simulink model "levitacao2"  (R2013a)
settings: Solver=FixedStepDiscrete  StartTime=0.0  StopTime=inf  RelTol=1e-3
undefined symbols (not defined in the file): DiscIntNeverNeededParam
libraries: arduino_io_lib x10, simulink x10
settings Model: Creator=gcampa  LastModifiedBy=Felipe
settings DataIOCC: SignalLoggingSaveFormat=ModelDataLogs
settings OptimizationCC: ExpressionDepthLimit=2147483647
settings DebuggingCC: FcnCallInpInsideContextMsg=UseLocalSettings
settings GRTTargetCC: CombineOutputUpdateFcns=off  GRTInterface=on

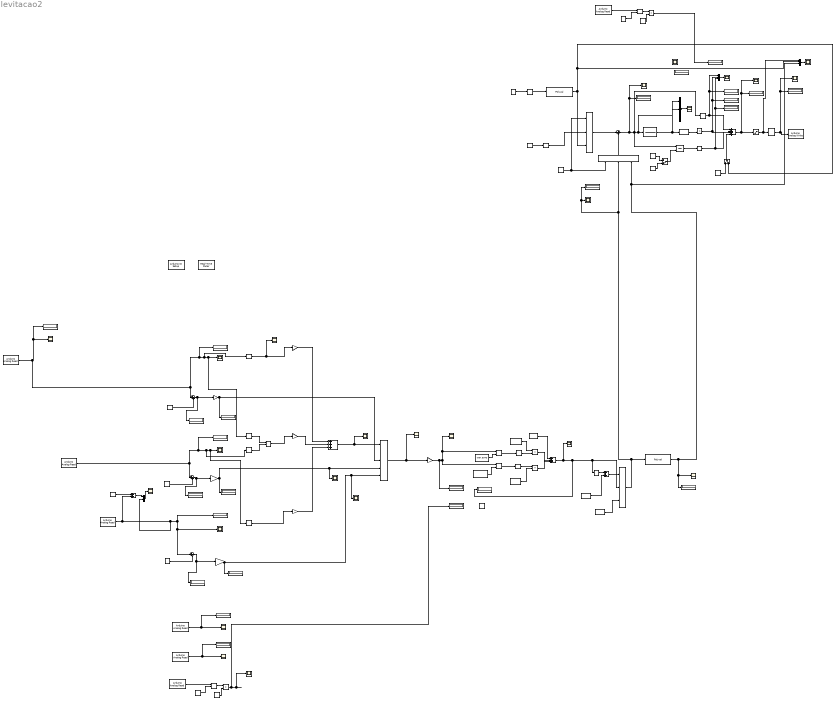
== system levitacao2 ==
  note: tem relacao com a distancia
  note: 0 para escolher realimentação do sinal de distancia cm
      | 1 para escolher sinal de realimentacao do sinal pwm0
  note: pwm0 ref
  note: funçao pwm0 X posicao(cm)
  note: bias - pwm0
  note: Funcao PWM0 X posicao0(cm)
  note: posicao em cm
  note: erro
  note: Set point ou distancia desejada em cm
  note: Distancia em cm
  note: Lê o potenciometro e envia para a saida pwm
  note: Sinal dos 3 sensores em 1 - sinal processado
  note: Converte sinal do sensor para distancia em cm - equação de decaimento exponencial de ordem 2
  note: se 1 - escolhe sensor 1
      | se 2 - escolhe sensor 2
      | se 3 - escolhe sensor 3
  note: Selecionando o sensor de acordo com sua sensibilidade para uma determinada faixa
  note: Tirando o ganho do amplificador
  note: Tirando o offset do circuito amplificador
  note: Tirando o offset do circuito amplificador
  note: Tirando o offset do circuito amplificador
  note: Tirando o ganho do amplificador
  note: Tirando o ganho do amplificador
  note: Selecionando o sensor de acordo com sua sensibilidade para uma determinada faixa
  note: Selecionando o sensor de acordo com sua sensibilidade para uma determinada faixa
  note: Set point ou distancia desejada em cm
  Add : Sum  Inputs=+++
  Add1 : Sum  Inputs=++++
  Add2 : Sum
  Arduino Analog Read16 : arduino_io_lib/Arduino Analog Read  arduinoVar=Temporary arduino variable: Arduino1  arduinoPin=1  T=0.00002
  Arduino Analog Read2 : arduino_io_lib/Arduino Analog Read  arduinoVar=Temporary arduino variable: Arduino1  arduinoPin=0  T=0.00002
  Arduino Analog Read3 : arduino_io_lib/Arduino Analog Read  arduinoVar=Temporary arduino variable: Arduino1  arduinoPin=3  T=0.00002
  Arduino Analog Read4 : arduino_io_lib/Arduino Analog Read  arduinoVar=Temporary arduino variable: Arduino1  arduinoPin=2  T=0.00002
  Arduino Analog Read5 : arduino_io_lib/Arduino Analog Read  arduinoVar=Temporary arduino variable: Arduino1  arduinoPin=2  T=0.001
  Arduino Analog Read6 : arduino_io_lib/Arduino Analog Read  arduinoVar=Temporary arduino variable: Arduino1  arduinoPin=4  T=0.01
  Arduino Analog Read7 : arduino_io_lib/Arduino Analog Read  arduinoVar=Temporary arduino variable: Arduino1  arduinoPin=3  T=0.001
  Arduino Analog Write3 : arduino_io_lib/Arduino Analog Write  arduinoVar=Temporary arduino variable: Arduino1  arduinoPin=5  T=0.00001
  Arduino IO Setup : arduino_io_lib/Arduino IO Setup  Priority=3  arduinoVar=Temporary arduino variable: Arduino1  workspaceVarName=a  comPort=COM3
  Compare To Constant : simulink/Logic and Bit Operations/Compare To Constant  relop=>=  const=56  OutDataTypeStr=boolean
  Compare To Constant1 : simulink/Logic and Bit Operations/Compare To Constant  relop=<  const=56  OutDataTypeStr=boolean
  Compare To Constant2 : simulink/Logic and Bit Operations/Compare To Constant  relop=>=  const=165  OutDataTypeStr=boolean
  Compare To Constant3 : simulink/Logic and Bit Operations/Compare To Constant  relop=<  const=160  OutDataTypeStr=boolean
  Compare To Constant4 : simulink/Logic and Bit Operations/Compare To Constant  relop=>  const=4  OutDataTypeStr=boolean
  Constant10 : Constant  Value=3.96648
  Constant11 : Constant  Value=0.01226
  Constant12 : Constant  Value=-56.90857
  Constant{9,13..16} (5 alike) : Constant
  Constant17 : Constant  Value=0
  Constant18 : Constant  Value=10
  Constant19 : Constant  Value=0
  Constant2 : Constant  Value=100
  Constant20 : Constant  Value=4
  Constant21 : Constant  Value=1023
  Constant22 : Constant  Value=0
  Constant23 : Constant  Value=0.00001
  Constant3 : Constant  Value=5
  Constant4 : Constant  Value=400
  Constant5 : Constant  Value=1023
  Constant6 : Constant  Value=256
  Constant7 : Constant  Value=2.24554
  Constant8 : Constant  Value=-587.5943
  Discrete Derivative : simulink/Discrete/Discrete Derivative  gainval=1.0  ICPrevScaledInput=0.0  InputProcessing=Inherited  OutMin=[]  OutMax=[]  OutDataType=fixdt(1, 16)  OutScaling=2^-10  DoSatur=off
  Discrete Filter1 : DiscreteFilter  Numerator=[0.5 0.5]  Denominator=[1 0.00001]  InputProcessing=Columns as channels (frame based)  FilterStructure=Direct form II transposed  a0EqualsOne=on
  Discrete-Time Integrator : DiscreteIntegrator  ExternalReset=either  SampleTime=0.00002  ICPrevOutput=DiscIntNeverNeededParam  ICPrevScaledInput=DiscIntNeverNeededParam
  Display{,1..24} (25 alike) : Display
  Divide{,1..3} (4 alike) : Product  Inputs=*/
  Gain : Gain
  Gain1 : Gain  Gain=2
  Gain2 : Gain  Gain=3
  Gain3 : Gain
  Gain4 : Gain  Gain=0.094
  Gain5 : Gain  Gain=0.024
  Gain6 : Gain  Gain=10
  Logical Operator : Logic  AllPortsSameDT=off  OutDataTypeStr=boolean
  Manual Switch : ManualSwitch  CurrentSetting=0
  Manual Switch1 : ManualSwitch  CurrentSetting=0
  Math Function : Math  SaturateOnIntegerOverflow=on
  Math Function1 : Math  SaturateOnIntegerOverflow=on
  Mode Multiport Switch : MultiPortSwitch  DataPortOrder=Zero-based contiguous  Inputs=4  zeroidx=on
  Mode Multiport Switch1 : MultiPortSwitch  DataPortOrder=Zero-based contiguous  Inputs=2  zeroidx=on
  Mode Multiport Switch2 : MultiPortSwitch  DataPortOrder=Zero-based contiguous  Inputs=2  zeroidx=on
  Mode Multiport Switch3 : MultiPortSwitch  DataPortOrder=Zero-based contiguous  Inputs=2  zeroidx=on
  Mux1 : Mux
      settings: DisplayOption=signals
  Mux2 : Mux  Inputs=2
      settings: DisplayOption=signals
  Mux3 : Mux
      settings: DisplayOption=signals
  Mux4 : Mux  Inputs=3
      settings: DisplayOption=signals
  Polynomial : Polyval  Coefs=[11.55, 16.03, 27.7 ]
  Polynomial1 : Polyval  Coefs=[11.55, 16.03, 27.7 ]
  Product{,1,3..5} (5 alike) : Product
  Rate Transition : RateTransition
  Real-Time Pacer : arduino_io_lib/Real-Time Pacer  simTimePerRealTime=1
  Saturation : Saturate  UpperLimit=255  LowerLimit=0
      settings: AttributesFormatString=max = %<UpperLimit>\nmin = %<LowerLimit>
  Scope{1..24} (24 alike) : Scope
      Scope1 settings: YMin=41  YMax=43.2
      Scope10 settings: YMin=0  YMax=1023  SaveName=ScopeData10
      Scope11 settings: YMin=4.25  YMax=8  SaveName=ScopeData11
      Scope12 settings: YMin=0  YMax=1023  SaveName=ScopeData12
      Scope13 settings: YMin=0  YMax=1023  SaveName=ScopeData13
      Scope14 settings: TimeRange=1  YMin=1  YMax=6.25  SaveName=ScopeData14
      Scope15 settings: YMin=-6  YMax=2  SaveName=ScopeData15
      Scope16 settings: TimeRange=0.1  YMin=80  YMax=155  SaveName=ScopeData16
      Scope17 settings: YMin=170.66  YMax=170.66  SaveName=ScopeData17
      Scope18 settings: TimeRange=1e-05  YMin=-75  YMax=250  SaveName=ScopeData18
      Scope19 settings: YMin=50  YMax=1100  SaveName=ScopeData19
      Scope2 settings: YMin=0  YMax=1023  SaveName=ScopeData2
      Scope20 settings: TimeRange=0.3  YMin=0  YMax=275  SaveName=ScopeData20
      Scope21 settings: TimeRange=1e-05  YMin=320  YMax=550  SaveName=ScopeData21
      Scope22 settings: YMin=2.5  YMax=50  SaveName=ScopeData22
      Scope23 settings: TimeRange=0.05  YMin=0  YMax=300  SaveName=ScopeData23
      Scope24 settings: TimeRange=0.01  YMin=0  YMax=180  SaveName=ScopeData24
      Scope3 settings: YMin=0  YMax=1023  SaveName=ScopeData3
      Scope4 settings: YMin=0  YMax=1023  SaveName=ScopeData4
      Scope5 settings: YMin=0  YMax=1023  SaveName=ScopeData5
      Scope6 settings: YMin=0  YMax=1023  SaveName=ScopeData6
      Scope7 settings: YMin=0  YMax=1023  SaveName=ScopeData7
      Scope8 settings: YMin=0  YMax=1023  SaveName=ScopeData8
      Scope9 settings: TimeRange=1  YMin=-2.5  YMax=27.5  SaveName=ScopeData9
  Slider Gain2 : simulink/Math Operations/Slider Gain  low=0  gain=2.5  high=3.6
  Slider Gain3 : simulink/Math Operations/Slider Gain  low=0  gain=1.24  high=2
  Slider Gain5 : simulink/Math Operations/Slider Gain  low=0  gain=0  high=100
  Slider Gain6 : simulink/Math Operations/Slider Gain  low=0  gain=2  high=3.6
  Subtract : Sum  Inputs=+++
  Subtract1 : Sum
  Sum : Sum  Inputs=|+-
  Sum1 : Sum  Inputs=|+-
  Sum2 : Sum  Inputs=|+-
  Sum3 : Sum  Inputs=|-+
  wires:
  Arduino Analog Read5/1 -> Display3/1, Scope4/1
  Arduino Analog Read6/1 -> Display4/1, Scope5/1
  Arduino Analog Read7/1 -> Divide/1
  Compare To Constant1/1 -> Logical Operator/1
  Compare To Constant2/1 -> Logical Operator/2
  Compare To Constant/1 -> Scope8/1, Gain/1
  Logical Operator/1 -> Gain1/1
  Compare To Constant3/1 -> Gain2/1
  Add/1 -> Mode Multiport Switch/1, Scope7/1
  Gain/1 -> Add/1
  Gain1/1 -> Add/2
  Gain2/1 -> Add/3
  Sum/1 -> Display10/1, Gain3/1
  Sum1/1 -> Display9/1, Gain4/1
  Sum2/1 -> Display11/1, Gain5/1
  Gain3/1 -> Mode Multiport Switch/3, Display6/1
  Gain4/1 -> Scope12/1, Mode Multiport Switch/4, Display7/1
  Gain5/1 -> Scope13/1, Mode Multiport Switch/5, Display8/1
  Mode Multiport Switch/1 -> Gain6/1, Scope9/1
  Constant2/1 -> Sum1/2
  Constant3/1 -> Sum/2
  Constant4/1 -> Sum2/2
  Constant5/1 -> Divide/2
  Divide/1 -> Product/1
  Constant6/1 -> Product/2
  Product/1 -> Display5/1, Scope6/1
  Constant12/1 -> Divide2/2
  Constant8/1 -> Divide1/2
  Divide2/1 -> Math Function/1
  Divide1/1 -> Math Function1/1
  Math Function1/1 -> Product3/2
  Math Function/1 -> Product4/1
  Constant7/1 -> Product3/1
  Constant10/1 -> Product4/2
  Product4/1 -> Subtract/3
  Product3/1 -> Subtract/2
  Constant11/1 -> Subtract/1
  Gain6/1 -> Display12/1, Divide1/1, Scope10/1, Divide2/1
  Constant13/1 -> Slider Gain2/1
  Slider Gain3/1 -> Display15/1, Mux1/1, Add1/1
  Slider Gain5/1 -> Display21/1, Mux1/3, Add1/3
  Add1/1 -> Saturation/1, Display17/1, Scope16/1
  Saturation/1 -> Mux3/1, Rate Transition/1
  Discrete-Time Integrator/1 -> Slider Gain5/1
  Mux1/1 -> Scope18/1
  Product5/1 -> Add1/2, Display20/1, Mux1/2
  Polynomial/1 -> Mode Multiport Switch2/3, Mux3/3, Display19/1, Scope19/1
  Constant14/1 -> Slider Gain6/1
  Slider Gain6/1 -> Polynomial1/1
  Mode Multiport Switch1/1 -> Sum3/1
  Constant15/1 -> Mode Multiport Switch2/1, Mode Multiport Switch1/1
  Mode Multiport Switch2/1 -> Sum3/2
  Manual Switch/1 -> Discrete-Time Integrator/2
  Constant16/1 -> Manual Switch/1
  Constant17/1 -> Manual Switch/2
  Slider Gain2/1 -> Mode Multiport Switch1/2
  Subtract/1 -> Scope11/1, Compare To Constant4/1, Mode Multiport Switch3/2, Display13/1
  Mux2/1 -> Scope21/1
  Add2/1 -> Mux2/1
  Constant18/1 -> Add2/1
  Manual Switch1/1 -> Add1/4
  Constant22/1 -> Manual Switch1/1
  Rate Transition/1 -> Display22/1, Scope20/1, Arduino Analog Write3/1
  Polynomial1/1 -> Mode Multiport Switch1/3, Manual Switch1/2, Mux3/2
  Compare To Constant4/1 -> Subtract1/1
  Mode Multiport Switch3/1 -> Display16/1, Scope14/1, Mode Multiport Switch2/2, Polynomial/1
  Constant19/1 -> Subtract1/2
  Subtract1/1 -> Mode Multiport Switch3/1
  Constant20/1 -> Mode Multiport Switch3/3
  Mux4/1 -> Scope24/1
  Arduino Analog Read3/1 -> Divide3/1
  Constant21/1 -> Divide3/2
  Divide3/1 -> Product1/1
  Constant23/1 -> Product1/2
  Product1/1 -> Display24/1
  Mux3/1 -> Scope23/1
  Discrete Derivative/1 -> Product5/2
  Sum3/1 -> Display18/1, Scope17/1, Slider Gain3/1, Discrete Filter1/1, Mux4/1, Discrete-Time Integrator/1
  Arduino Analog Read16/1 -> Display1/1, Compare To Constant2/1, Compare To Constant3/1, Scope2/1, Sum1/1
  Arduino Analog Read4/1 -> Mux2/2, Sum2/1, Scope3/1, Display2/1, Add2/2
  Arduino Analog Read2/1 -> Sum/1, Display/1, Compare To Constant/1, Compare To Constant1/1, Scope1/1, Display23/1, Scope22/1
  Discrete Filter1/1 -> Mux4/2, Discrete Derivative/1
